simulink model "simulinkmich"  (R2014b)
settings: Solver=ode45  StartTime=0.0  StopTime=10.0  RelTol=1e-3
undefined symbols (not defined in the file): A, C_d, c_rr, g, G, ke, M, Qbatt, r_w, ro, Vbatt
libraries: simulink x3
settings Model: Creator=PC-MEK  LastModifiedBy=PC-MEK

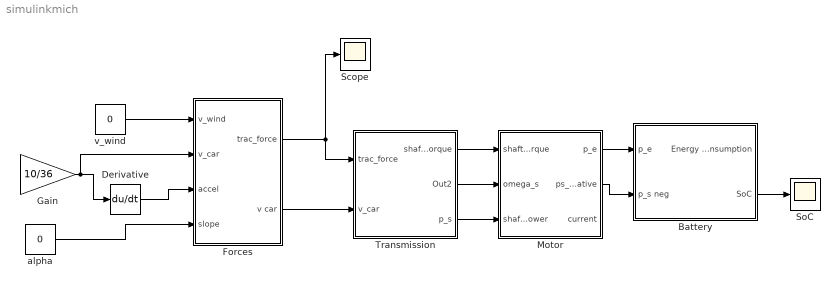
== system simulinkmich ==
  Battery : Subsystem
  Derivative : Derivative
  Forces : Subsystem
  Gain : Gain  Gain=10/36
  Motor : Subsystem
  Scope : Scope
  SoC : Scope
  Transmission : Subsystem
  alpha : Constant  Value=0
  v_wind : Constant  Value=0
  wires:
  Motor/1(p_e) -> Battery/1(p_e)
  Transmission/1(shaft_torque) -> Motor/1(shaft_torque)
  Forces/1(trac_force) -> Transmission/1(trac_force), Scope/1
  Forces/2(v car) -> Transmission/2(v_car)
  alpha/1 -> Forces/4(slope)
  Derivative/1 -> Forces/3(accel)
  Gain/1 -> Forces/2(v_car), Derivative/1
  v_wind/1 -> Forces/1(v_wind)
  Transmission/2(Out2) -> Motor/2(omega_s)
  Transmission/3(p_s) -> Motor/3(shaft_power)
  Motor/2(ps_negative) -> Battery/2(p_s neg)
  Battery/2(SoC) -> SoC/1

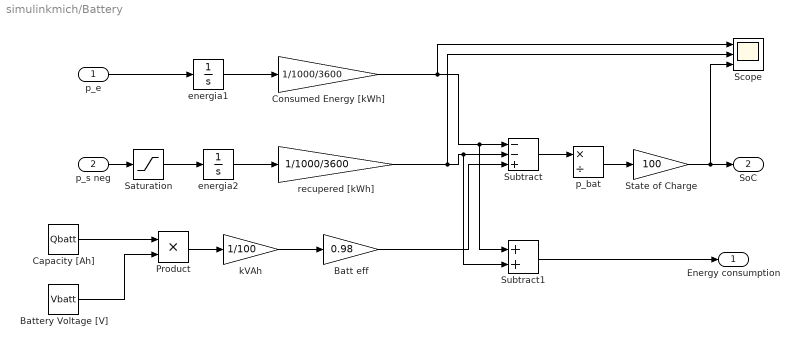
== system simulinkmich/Battery ==
  p_e : Inport
  p_s neg : Inport  Port=2
  Batt eff : Gain  Gain=0.98
  Battery Voltage [V] : Constant  Value=Vbatt
  Capacity [Ah] : Constant  Value=Qbatt
  Consumed Energy [kWh] : Gain  Gain=1/1000/3600
  Product : Product
  Saturation : Saturate
  Scope : Scope  NumInputPorts=3
      settings: YMin=-5~-5~-5  YMax=5~5~5  SaveName=ScopeData5
  State of Charge : Gain  Gain=100
  Subtract : Sum  Inputs=--+
  Subtract1 : Sum
  energia1 : Integrator
  energia2 : Integrator
  kVAh : Gain  Gain=1/100
  p_bat : Product  Inputs=*/
  recupered [kWh] : Gain  Gain=1/1000/3600
  Energy consumption : Outport
  SoC : Outport  Port=2
  wires:
  State of Charge/1 -> Scope/3, SoC/1
  p_bat/1 -> State of Charge/1
  Capacity [Ah]/1 -> Product/1
  Battery Voltage [V]/1 -> Product/2
  Product/1 -> kVAh/1
  kVAh/1 -> Batt eff/1
  Subtract/1 -> p_bat/1
  p_e/1 -> energia1/1
  p_s neg/1 -> Saturation/1
  Saturation/1 -> energia2/1
  energia2/1 -> recupered [kWh]/1
  energia1/1 -> Consumed Energy [kWh]/1
  Consumed Energy [kWh]/1 -> Scope/1, Subtract1/1, Subtract/1
  recupered [kWh]/1 -> Scope/2, Subtract1/2, Subtract/2
  Batt eff/1 -> Subtract/3
  Subtract1/1 -> Energy consumption/1

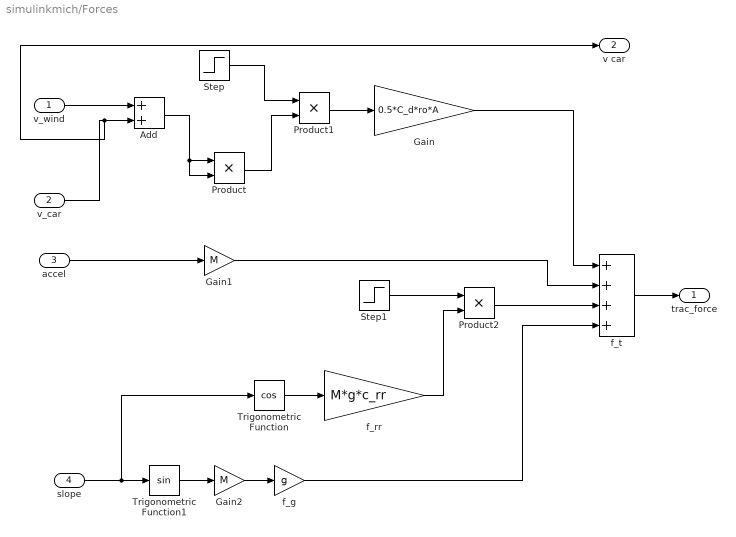
== system simulinkmich/Forces ==
  v_wind : Inport
  v_car : Inport  Port=2
  accel : Inport  Port=3
  slope : Inport  Port=4
  Add : Sum
  Gain : Gain  Gain=0.5*C_d*ro*A
  Gain1 : Gain  Gain=M
  Gain2 : Gain  Gain=M
  Product : Product
  Product1 : Product
  Product2 : Product
  Step : Step  SampleTime=0
  Step1 : Step  SampleTime=0
  Trigonometric Function : Trigonometry  Operator=cos
  Trigonometric Function1 : Trigonometry
  f_g : Gain  Gain=g
  f_rr : Gain  Gain=M*g*c_rr
  f_t : Sum  Inputs=++++
  trac_force : Outport
  v car : Outport  Port=2
  wires:
  Product1/1 -> Gain/1
  Product/1 -> Product1/2
  Step/1 -> Product1/1
  Add/1 -> Product/1, Product/2
  v_wind/1 -> Add/1
  v_car/1 -> v car/1, Add/2
  f_t/1 -> trac_force/1
  Trigonometric Function/1 -> f_rr/1
  Gain2/1 -> f_g/1
  Trigonometric Function1/1 -> Gain2/1
  slope/1 -> Trigonometric Function/1, Trigonometric Function1/1
  f_g/1 -> f_t/4
  Product2/1 -> f_t/3
  f_rr/1 -> Product2/2
  Step1/1 -> Product2/1
  accel/1 -> Gain1/1
  Gain1/1 -> f_t/2
  Gain/1 -> f_t/1

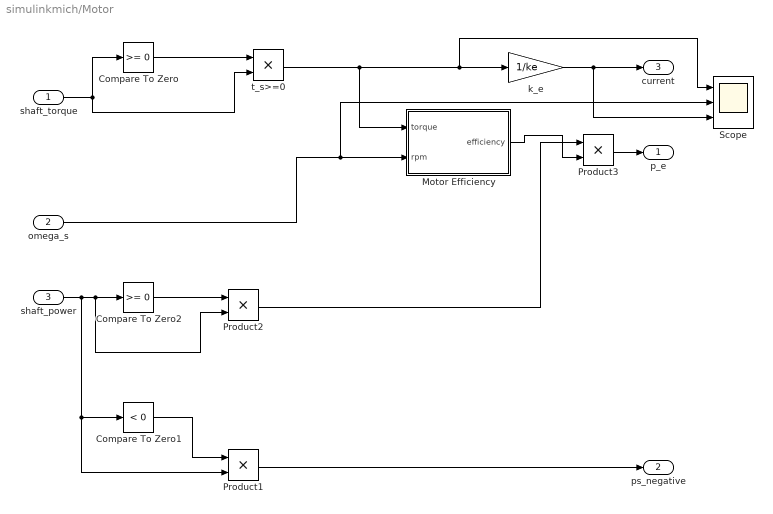
== system simulinkmich/Motor ==
  shaft_torque : Inport
  omega_s : Inport  Port=2
  shaft_power : Inport  Port=3
  Compare To Zero : simulink/Logic and Bit Operations/Compare To Zero  relop=>=  OutDataTypeStr=boolean
  Compare To Zero1 : simulink/Logic and Bit Operations/Compare To Zero  relop=<  OutDataTypeStr=boolean
  Compare To Zero2 : simulink/Logic and Bit Operations/Compare To Zero  relop=>=  OutDataTypeStr=boolean
  Motor Efficiency : Subsystem
  Product1 : Product
  Product2 : Product
  Product3 : Product
  Scope : Scope  NumInputPorts=3
      settings: YMin=-5~-5~-5  YMax=5~5~5  SaveName=ScopeData4
  k_e : Gain  Gain=1/ke
  t_s>=0 : Product
  p_e : Outport
  ps_negative : Outport  Port=2
  current : Outport  Port=3
  wires:
  Compare To Zero/1 -> t_s>=0/1
  shaft_torque/1 -> Compare To Zero/1, t_s>=0/2
  k_e/1 -> Scope/3, current/1
  t_s>=0/1 -> Motor Efficiency/1(torque), Scope/1, k_e/1
  Product3/1 -> p_e/1
  omega_s/1 -> Scope/2, Motor Efficiency/2(rpm)
  Compare To Zero2/1 -> Product2/1
  Compare To Zero1/1 -> Product1/1
  shaft_power/1 -> Compare To Zero1/1, Product1/2, Product2/2, Compare To Zero2/1
  Product1/1 -> ps_negative/1
  Product2/1 -> Product3/1
  Motor Efficiency/1(efficiency) -> Product3/2

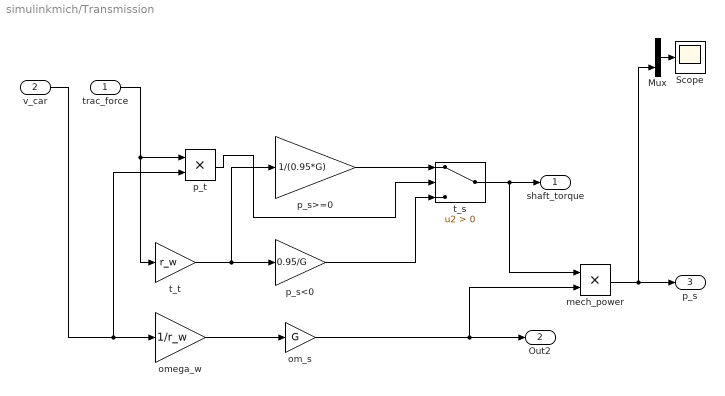
== system simulinkmich/Transmission ==
  trac_force : Inport
  v_car : Inport  Port=2
  Mux : Mux  Inputs=2
  Scope : Scope
      settings: SaveName=ScopeData2
  "mech_power " : Product
  om_s : Gain  Gain=G
  omega_w : Gain  Gain=1/r_w
  p_s<0 : Gain  Gain=0.95/G
  p_s>=0 : Gain  Gain=1/(0.95*G)
  p_t : Product
  t_s : Switch  Criteria=u2 > Threshold
  t_t : Gain  Gain=r_w
  shaft_torque : Outport
  Out2 : Outport  Port=2
  p_s : Outport  Port=3
  wires:
  Mux/1 -> Scope/1
  "mech_power "/1 -> Mux/2, p_s/1
  trac_force/1 -> t_t/1, p_t/1
  t_t/1 -> p_s>=0/1, p_s<0/1
  omega_w/1 -> om_s/1
  p_s>=0/1 -> t_s/1
  p_t/1 -> t_s/2
  p_s<0/1 -> t_s/3
  t_s/1 -> "mech_power "/1, shaft_torque/1
  om_s/1 -> "mech_power "/2, Out2/1
  v_car/1 -> p_t/2, omega_w/1

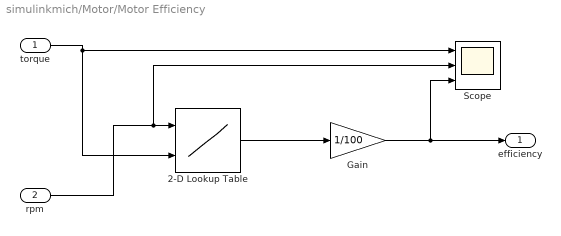
== system simulinkmich/Motor/Motor Efficiency ==
  torque : Inport
  rpm : Inport  Port=2
  2-D Lookup Table : Lookup_n-D  BreakpointsForDimension1=[1:3]  BreakpointsForDimension2=[1:3]  InternalRulePriority=Speed  RndMeth=Simplest  InputSameDT=on
  Gain : Gain  Gain=1/100
  Scope : Scope  NumInputPorts=3
      settings: YMin=-5~-5~-5  YMax=5~5~5  SaveName=ScopeData3
  efficiency : Outport
  wires:
  rpm/1 -> Scope/2, 2-D Lookup Table/1
  torque/1 -> Scope/1, 2-D Lookup Table/2
  2-D Lookup Table/1 -> Gain/1
  Gain/1 -> Scope/3, efficiency/1
